simulink model "Sim_AdaptiveFinalazo_ultimo2012a"  (R2012a)
settings: Solver=ode45  SolverMode=SingleTasking  StartTime=0.0  StopTime=10.0  RelTol=1e-3
values from neighbouring files (symbols this model uses):
  In = 0.002381    [parametros_ultimo.m]
  Kn = 0.0347    [parametros_ultimo.m]
  Ln = 0.2175    [parametros_ultimo.m]
  Mn = 0.1047708    [parametros_ultimo.m]
settings Model: Creator=Harryth  LastModifiedBy=i95sa
settings DataIOCC: LimitDataPoints=on  SaveFormat=Array  ReturnWorkspaceOutputs=off
settings OptimizationCC: BlockReduction=off  BooleanDataType=off  LifeSpan=inf  SimCompilerOptimization=Off
settings DebuggingCC: SaveWithParameterizedLinksMsg=none  UnderspecifiedInitializationDetection=Classic  MergeDetectMultiDrivingBlocksExec=none  SignalResolutionControl=TryResolveAllWithWarning  FcnCallInpInsideContextMsg=Enable All  SFUnexpectedBacktrackingDiag=warning  SFNoUnconditionalDefaultTransitionDiag=warning
settings HardwareCC: ProdBitPerPointer=32  ProdLargestAtomicFloat=None  ProdIntDivRoundTo=Undefined  ProdEndianess=Unspecified  ProdWordSize=32  ProdHWDeviceType=32-bit Generic  TargetUnknown=on
settings ModelReferenceCC: PropagateSignalLabelsOutOfModel=off
settings SFSimCC: SimUseLocalCustomCode=off
settings RTWCC: RTWUseLocalCustomCode=off  RTWCompilerOptimization=Off
settings GRTTargetCC: CodeReplacementLibrary=C89/C90 (ANSI)  GeneratePreprocessorConditionals=Disable all  CPPClassGenCompliant=off

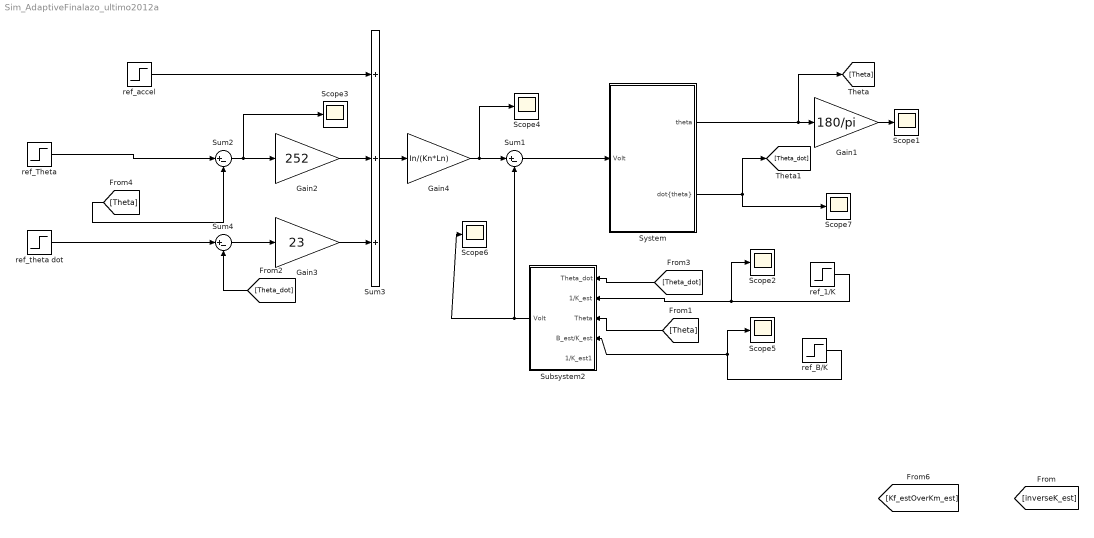
== system Sim_AdaptiveFinalazo_ultimo2012a ==
  Gain1 : Gain  Gain=180/pi
  Gain2 : Gain  Gain=252
  Gain3 : Gain  Gain=23
  Gain4 : Gain  Gain=In/(Kn*Ln)
  Scope{1..7} (7 alike) : Scope
      Scope1 settings: TimeRange=auto  MaxDataPoints=5000  SaveName=x1  YMin=-60.96258  YMax=176.24064  SampleTime=-1  DataFormat=Array
      Scope2 settings: TimeRange=auto  LimitDataPoints=on  MaxDataPoints=5000  SaveToWorkspace=off  SaveName=ScopeData  YMin=-10  YMax=10  SampleTime=-1  DataFormat=Array
      Scope3 settings: TimeRange=auto  LimitDataPoints=on  MaxDataPoints=5000  SaveToWorkspace=off  SaveName=ScopeData  YMin=-10  YMax=10  SampleTime=-1  DataFormat=Array
      Scope4 settings: TimeRange=auto  LimitDataPoints=on  MaxDataPoints=5000  SaveToWorkspace=off  SaveName=ScopeData  YMin=-10  YMax=10  SampleTime=-1  DataFormat=Array
      Scope5 settings: TimeRange=auto  LimitDataPoints=on  MaxDataPoints=5000  SaveToWorkspace=off  SaveName=ScopeData  YMin=-10  YMax=10  SampleTime=-1  DataFormat=Array
      Scope6 settings: TimeRange=auto  LimitDataPoints=on  MaxDataPoints=5000  SaveToWorkspace=off  SaveName=ScopeData  YMin=-10  YMax=10  SampleTime=-1  DataFormat=Array
      Scope7 settings: TimeRange=auto  MaxDataPoints=5000  SaveName=x  YMin=-0.646  YMax=5.76289  SampleTime=-1  DataFormat=Array
  Subsystem2 : Subsystem
  Sum1 : Sum  Inputs=|+-
  Sum2 : Sum  Inputs=|+-
  Sum3 : Sum  Inputs=+++
  Sum4 : Sum  Inputs=|+-
  System : Subsystem
  ref_1/K : Step  Time=0  After=1/0.0347  SampleTime=0
  ref_B/K : Step  Time=0  After=0.0055/0.0347  SampleTime=0
  ref_Theta : Step  Time=0  After=pi/2  SampleTime=0
  ref_accel : Step  Time=0  After=0  SampleTime=0
  ref_theta dot : Step  Time=0  After=0  SampleTime=0
  wires:
  System/2("dot{theta}") -> Scope7/1, [Theta_dot]
  Sum1/1 -> System/1(Volt)
  Subsystem2/1(Volt) -> Scope6/1, Sum1/2
  ref_accel/1 -> Sum3/1
  ref_1/K/1 -> Scope2/1, Subsystem2/2(1/K_est)
  [Theta] -> Subsystem2/3(Theta)
  [Theta_dot] -> Subsystem2/1(Theta_dot)
  ref_B/K/1 -> Subsystem2/4(B_est/K_est), Scope5/1
  System/1(theta) -> Gain1/1, [Theta]
  Gain1/1 -> Scope1/1
  Sum2/1 -> Scope3/1, Gain2/1
  [Theta] -> Sum2/2
  Sum4/1 -> Gain3/1
  [Theta_dot] -> Sum4/2
  Gain2/1 -> Sum3/2
  Gain3/1 -> Sum3/3
  ref_Theta/1 -> Sum2/1
  ref_theta dot/1 -> Sum4/1
  Sum3/1 -> Gain4/1
  Gain4/1 -> Scope4/1, Sum1/1

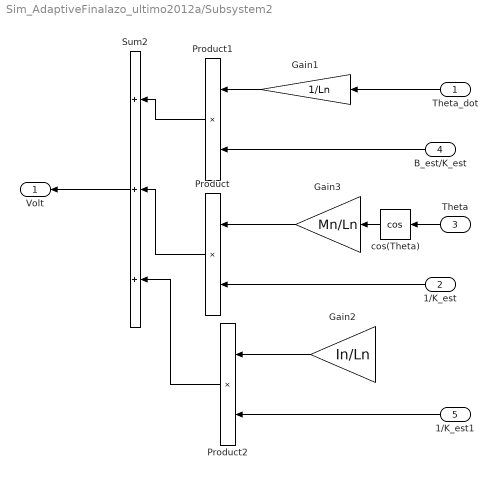
== system Sim_AdaptiveFinalazo_ultimo2012a/Subsystem2 ==
  Theta_dot : Inport
  1/K_est : Inport  Port=2
  Theta : Inport  Port=3
  B_est/K_est : Inport  Port=4
  1/K_est1 : Inport  Port=5
  Gain1 : Gain  Gain=1/Ln
  Gain2 : Gain  Gain=In/Ln
  Gain3 : Gain  Gain=Mn/Ln
  Product : Product  RndMeth=Zero
  Product1 : Product  RndMeth=Zero
  Product2 : Product  RndMeth=Zero
  Sum2 : Sum  Inputs=+++
  cos(Theta) : Trigonometry  Operator=cos
  Volt : Outport
  wires:
  cos(Theta)/1 -> Gain3/1
  Gain3/1 -> Product/1
  Product/1 -> Sum2/2
  Theta_dot/1 -> Gain1/1
  Theta/1 -> cos(Theta)/1
  Sum2/1 -> Volt/1
  1/K_est/1 -> Product/2
  Gain1/1 -> Product1/1
  Product1/1 -> Sum2/1
  B_est/K_est/1 -> Product1/2
  ? -> Gain2/1
  Gain2/1 -> Product2/1
  Product2/1 -> Sum2/3
  1/K_est1/1 -> Product2/2

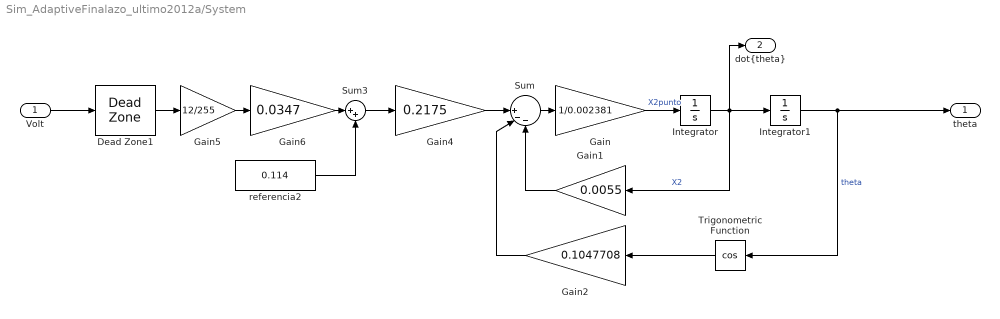
== system Sim_AdaptiveFinalazo_ultimo2012a/System ==
  Volt : Inport
  Dead Zone1 : DeadZone  LowerValue=0  UpperValue=0  SaturateOnIntegerOverflow=on
  Gain : Gain  Gain=1/0.002381
  Gain1 : Gain  Gain=0.0055
  Gain2 : Gain  Gain=0.1047708
  Gain4 : Gain  Gain=0.2175
  Gain5 : Gain  Gain=12/255
  Gain6 : Gain  Gain=0.0347
  Integrator : Integrator
  Integrator1 : Integrator  InitialCondition=-0.65
  Sum : Sum  Inputs=||+--
  Sum3 : Sum  Inputs=|++
  Trigonometric Function : Trigonometry  Operator=cos
  referencia2 : Constant  Value=0.114
  theta : Outport
  "dot{theta}" : Outport  Port=2
  wires:
  Sum/1 -> Gain/1
  Gain/1 -> Integrator/1  "X2punto"
  Integrator/1 -> "dot{theta}"/1, Integrator1/1, Gain1/1  "X2"
  Trigonometric Function/1 -> Gain2/1
  Gain1/1 -> Sum/3
  Integrator1/1 -> Trigonometric Function/1, theta/1  "theta"
  Gain2/1 -> Sum/2
  Gain4/1 -> Sum/1
  referencia2/1 -> Sum3/2
  Sum3/1 -> Gain4/1
  Gain5/1 -> Gain6/1
  Gain6/1 -> Sum3/1
  Dead Zone1/1 -> Gain5/1
  Volt/1 -> Dead Zone1/1
